simulink model "COSTEP_Exergy"  (R2024b)
settings: Solver=FixedStepAuto  StartTime=0.0  StopTime=25  FixedStep=1/3600  RelTol=1e-3
model workspace (MAT data in the model file):
  AD : Simulink.Parameter (value not decoded)
  AG : Simulink.Parameter (value not decoded)
  AH : Simulink.Parameter (value not decoded)
  AV : Simulink.Parameter (value not decoded)
  AVP : Simulink.Parameter (value not decoded)
  BCHL : Simulink.Parameter (value not decoded)
  BCHV : Simulink.Parameter (value not decoded)
  BD : Simulink.Parameter (value not decoded)
  BDIST : Simulink.Parameter (value not decoded)
  BG : Simulink.Parameter (value not decoded)
  BH : Simulink.Parameter (value not decoded)
  BVP : Simulink.Parameter (value not decoded)
  CD : Simulink.Parameter (value not decoded)
  CDIST : Simulink.Parameter (value not decoded)
  CG : Simulink.Parameter (value not decoded)
  CH : Simulink.Parameter (value not decoded)
  CVP : Simulink.Parameter (value not decoded)
  DDIST : Simulink.Parameter (value not decoded)
  DIST_CONST : Simulink.Parameter (value not decoded)
  ISV : Simulink.Parameter (value not decoded)
  TLAST : Simulink.Parameter (value not decoded)
  TNEXT : Simulink.Parameter (value not decoded)
  XMW : Simulink.Parameter (value not decoded)
  XNS : Simulink.Parameter (value not decoded)
  XNS2 : Simulink.Parameter (value not decoded)
  XNS3 : Simulink.Parameter (value not decoded)
  XNSADD : Simulink.Parameter (value not decoded)
  XNSE : Simulink.Parameter (value not decoded)
symbols that are objects in the model workspace (value not decoded): AD, AG, AH, AV, AVP, BD, BG, BH, BVP, CD, CG, CH, CVP, XMW, XNS, XNS2, XNS3, XNSE
undefined symbols (not defined in the file or in its folder): magnitude, msgbox, SETPT, XMEAS, XMV
libraries: mylib x403, dspindex x31
(part 10 of 13)

== system COSTEP_Exergy/Subsystem1/Condenser cooling water/CCin/Subsystem3 ==
  TC : Inport
  Add : Sum  Inputs=+-
  P Water Vapour Pressure Pa : Subsystem
  P0 Pa : Constant  Value=1.01325e5
  Subsystem : Subsystem
  Subsystem1 : Subsystem
  Subsystem2 : Subsystem
  T0 K : Constant  Value=298.15
  Bph : Outport
  wires:
  P Water Vapour Pressure Pa/1(P) -> Subsystem1/3(P1)
  P0 Pa/1 -> Subsystem1/4(P0)
  Subsystem/1(h-h0 J/mol) -> Add/1
  Subsystem1/1(T0(s-s0) J/mol) -> Add/2
  T0 K/1 -> Subsystem1/2(T0), Subsystem/2(T0)
  Subsystem2/1(TK) -> Subsystem/1(T1), Subsystem1/1(T1), P Water Vapour Pressure Pa/1(TK)
  TC/1 -> Subsystem2/1(TC)
  Add/1 -> Bph/1

== system COSTEP_Exergy/Subsystem1/Condenser cooling water/CCout/Subsystem ==
  Bph : Inport
  FWS : Inport  Port=2
  Gain : Gain  Gain=1/3600
  Product : Product
  Product1 : Product
  gpm to lb/h : Constant  Value=500.72
  lb/h to lb-mol/h : Product  Inputs=*/
  lb/lb-mol : Constant  Value=18.02
  mol : Constant  Value=453.59
  mol/h : Product
  Bphm J/s : Outport  VectorParamsAs1DForOutWhenUnconnected=off
  wires:
  Product/1 -> Gain/1
  mol/1 -> mol/h/1
  mol/h/1 -> Product/2
  Bph/1 -> Product/1
  FWS/1 -> Product1/1
  gpm to lb/h/1 -> Product1/2
  Product1/1 -> lb/h to lb-mol/h/1
  lb/h to lb-mol/h/1 -> mol/h/2
  lb/lb-mol/1 -> lb/h to lb-mol/h/2
  Gain/1 -> Bphm J/s/1

== system COSTEP_Exergy/Subsystem1/Condenser cooling water/CCout/Subsystem1 ==
  T : Inport
  F : Inport  Port=2
  A : Constant  Value=9.069
  Gain : Gain  Gain=1/3600
  J/mol : Product
  Product : Product
  Product1 : Product
  gpm to lb/h : Constant  Value=500.72
  lb/h to lb-mol/h : Product  Inputs=*/
  lb/lb-mol : Constant  Value=18.02
  mol : Constant  Value=453.59
  mol/h : Product
  Q J/s : Outport  VectorParamsAs1DForOutWhenUnconnected=off
  wires:
  A/1 -> J/mol/1
  mol/1 -> mol/h/1
  lb/lb-mol/1 -> lb/h to lb-mol/h/2
  Product1/1 -> lb/h to lb-mol/h/1
  lb/h to lb-mol/h/1 -> mol/h/2
  Product/1 -> Gain/1
  gpm to lb/h/1 -> Product1/2
  Gain/1 -> Q J/s/1
  mol/h/1 -> Product/2
  J/mol/1 -> Product/1
  T/1 -> J/mol/2
  F/1 -> Product1/1

== system COSTEP_Exergy/Subsystem1/Condenser cooling water/CCout/Subsystem3 ==
  TC : Inport
  Add : Sum  Inputs=+-
  P Water Vapour Pressure Pa : Subsystem
  P0 Pa : Constant  Value=1.01325e5
  Subsystem : Subsystem
  Subsystem1 : Subsystem
  Subsystem2 : Subsystem
  T0 K : Constant  Value=298.15
  Bph : Outport
  wires:
  P Water Vapour Pressure Pa/1(P) -> Subsystem1/3(P1)
  P0 Pa/1 -> Subsystem1/4(P0)
  Subsystem/1(h-h0 J/mol) -> Add/1
  Subsystem1/1(T0(s-s0) J/mol) -> Add/2
  T0 K/1 -> Subsystem1/2(T0), Subsystem/2(T0)
  Subsystem2/1(TK) -> Subsystem/1(T1), Subsystem1/1(T1), P Water Vapour Pressure Pa/1(TK)
  TC/1 -> Subsystem2/1(TC)
  Add/1 -> Bph/1

== system COSTEP_Exergy/Subsystem1/Reactor cooling water/RCin/Subsystem ==
  Bph : Inport
  FWR : Inport  Port=2
  Gain : Gain  Gain=1/3600
  Product : Product
  Product1 : Product
  gpm to lb/h : Constant  Value=500.72
  lb/h to lb-mol/h : Product  Inputs=*/
  lb/lb-mol : Constant  Value=18.02
  mol : Constant  Value=453.59
  mol/h : Product
  Bphm J/s : Outport  VectorParamsAs1DForOutWhenUnconnected=off
  wires:
  Product/1 -> Gain/1
  mol/1 -> mol/h/1
  mol/h/1 -> Product/2
  Bph/1 -> Product/1
  FWR/1 -> Product1/1
  gpm to lb/h/1 -> Product1/2
  Product1/1 -> lb/h to lb-mol/h/1
  lb/h to lb-mol/h/1 -> mol/h/2
  lb/lb-mol/1 -> lb/h to lb-mol/h/2
  Gain/1 -> Bphm J/s/1

== system COSTEP_Exergy/Subsystem1/Reactor cooling water/RCin/Subsystem1 ==
  T : Inport
  F : Inport  Port=2
  A : Constant  Value=9.069
  Gain : Gain  Gain=1/3600
  J/mol : Product
  Product : Product
  Product1 : Product
  gpm to lb/h : Constant  Value=500.72
  lb/h to lb-mol/h : Product  Inputs=*/
  lb/lb-mol : Constant  Value=18.02
  mol : Constant  Value=453.59
  mol/h : Product
  Q J/s : Outport  VectorParamsAs1DForOutWhenUnconnected=off
  wires:
  A/1 -> J/mol/1
  mol/1 -> mol/h/1
  lb/lb-mol/1 -> lb/h to lb-mol/h/2
  Product1/1 -> lb/h to lb-mol/h/1
  lb/h to lb-mol/h/1 -> mol/h/2
  Product/1 -> Gain/1
  gpm to lb/h/1 -> Product1/2
  Gain/1 -> Q J/s/1
  mol/h/1 -> Product/2
  J/mol/1 -> Product/1
  T/1 -> J/mol/2
  F/1 -> Product1/1

== system COSTEP_Exergy/Subsystem1/Reactor cooling water/RCin/Subsystem3 ==
  TC : Inport
  Add : Sum  Inputs=+-
  P Water Vapour Pressure Pa : Subsystem
  P0 Pa : Constant  Value=1.01325e5
  Subsystem : Subsystem
  Subsystem1 : Subsystem
  Subsystem2 : Subsystem
  T0 K : Constant  Value=298.15
  Bph : Outport
  wires:
  P Water Vapour Pressure Pa/1(P) -> Subsystem1/3(P1)
  P0 Pa/1 -> Subsystem1/4(P0)
  Subsystem/1(h-h0 J/mol) -> Add/1
  Subsystem1/1(T0(s-s0) J/mol) -> Add/2
  T0 K/1 -> Subsystem1/2(T0), Subsystem/2(T0)
  Subsystem2/1(TK) -> Subsystem/1(T1), Subsystem1/1(T1), P Water Vapour Pressure Pa/1(TK)
  TC/1 -> Subsystem2/1(TC)
  Add/1 -> Bph/1

== system COSTEP_Exergy/Subsystem1/Reactor cooling water/RCout/Subsystem ==
  Bph : Inport
  FWR : Inport  Port=2
  Gain : Gain  Gain=1/3600
  Product : Product
  Product1 : Product
  gpm to lb/h : Constant  Value=500.72
  lb/h to lb-mol/h : Product  Inputs=*/
  lb/lb-mol : Constant  Value=18.02
  mol : Constant  Value=453.59
  mol/h : Product
  Bphm J/s : Outport  VectorParamsAs1DForOutWhenUnconnected=off
  wires:
  Product/1 -> Gain/1
  mol/1 -> mol/h/1
  mol/h/1 -> Product/2
  Bph/1 -> Product/1
  FWR/1 -> Product1/1
  gpm to lb/h/1 -> Product1/2
  Product1/1 -> lb/h to lb-mol/h/1
  lb/h to lb-mol/h/1 -> mol/h/2
  lb/lb-mol/1 -> lb/h to lb-mol/h/2
  Gain/1 -> Bphm J/s/1

== system COSTEP_Exergy/Subsystem1/Reactor cooling water/RCout/Subsystem1 ==
  T : Inport
  F : Inport  Port=2
  A : Constant  Value=9.069
  Gain : Gain  Gain=1/3600
  J/mol : Product
  Product : Product
  Product1 : Product
  gpm to lb/h : Constant  Value=500.72
  lb/h to lb-mol/h : Product  Inputs=*/
  lb/lb-mol : Constant  Value=18.02
  mol : Constant  Value=453.59
  mol/h : Product
  Q J/s : Outport  VectorParamsAs1DForOutWhenUnconnected=off
  wires:
  A/1 -> J/mol/1
  mol/1 -> mol/h/1
  lb/lb-mol/1 -> lb/h to lb-mol/h/2
  Product1/1 -> lb/h to lb-mol/h/1
  lb/h to lb-mol/h/1 -> mol/h/2
  Product/1 -> Gain/1
  gpm to lb/h/1 -> Product1/2
  Gain/1 -> Q J/s/1
  mol/h/1 -> Product/2
  J/mol/1 -> Product/1
  T/1 -> J/mol/2
  F/1 -> Product1/1

== system COSTEP_Exergy/Subsystem1/Reactor cooling water/RCout/Subsystem3 ==
  TC : Inport
  Add : Sum  Inputs=+-
  P Water Vapour Pressure Pa : Subsystem
  P0 Pa : Constant  Value=1.01325e5
  Subsystem : Subsystem
  Subsystem1 : Subsystem
  Subsystem2 : Subsystem
  T0 K : Constant  Value=298.15
  Bph : Outport
  wires:
  P Water Vapour Pressure Pa/1(P) -> Subsystem1/3(P1)
  P0 Pa/1 -> Subsystem1/4(P0)
  Subsystem/1(h-h0 J/mol) -> Add/1
  Subsystem1/1(T0(s-s0) J/mol) -> Add/2
  T0 K/1 -> Subsystem1/2(T0), Subsystem/2(T0)
  Subsystem2/1(TK) -> Subsystem/1(T1), Subsystem1/1(T1), P Water Vapour Pressure Pa/1(TK)
  TC/1 -> Subsystem2/1(TC)
  Add/1 -> Bph/1

== system COSTEP_Exergy/Control Mode/Braatz/ /CONTROL 14/PI Control Setpoint Velocity form ==
  Setpoint : Inport
  Measurement : Inport  Port=2
  Gain : Gain  Gain=H/100
  Subsystem : Subsystem  mask{Kc=Kc, Ti=Ti, Ts=Ts, HS=HS}
      mask prompts: Kc "Controller Gain - Kc"; Ti "Integral Time - Ti"; Ts "Sampling Interval - Ts"; HS "High limit of setpoint"
      mask DialogControl DescGroupVar Prompt: Control Parameters
  Sum : Sum  Inputs=|++  SaturateOnIntegerOverflow=on
  Unit Delay : UnitDelay  InitialCondition=X_0  SampleTime=Ts
  Output : Outport
  wires:
  Gain/1 -> Sum/1
  Subsystem/1(Delta Output) -> Gain/1
  Measurement/1 -> Subsystem/2(Measurement)
  Setpoint/1 -> Subsystem/1(Setpoint)
  Sum/1 -> Unit Delay/1, Output/1
  Unit Delay/1 -> Sum/2

== system COSTEP_Exergy/Control Mode/Braatz/ 10/CONTROL 6/P Control Velocity form ==
  Setpoint : Inport
  Measurement : Inport  Port=2
  XMEAS : Inport  Port=3
  Pressure limits : Subsystem
      mask Display: color('Blue'),disp('Pressure limits'),
  Subsystem : Subsystem  mask{Kc=Kc, Ts=Ts, H=H}
      mask prompts: Kc "Controller Gain - Kc"; Ts "Sampling Interval - Ts"; H "High limit of measurement"
      mask DialogControl DescGroupVar Prompt: Control Parameters
  Sum : Sum  Inputs=|++  SaturateOnIntegerOverflow=on
  Unit Delay : UnitDelay  InitialCondition=X_0  SampleTime=Ts
  Output : Outport
  wires:
  Unit Delay/1 -> Output/1, Sum/2
  Sum/1 -> Pressure limits/1("XMV(6) ")
  Setpoint/1 -> Subsystem/1(Setpoint)
  Pressure limits/1(XMV(6)) -> Unit Delay/1
  Subsystem/1(Delta Output) -> Sum/1
  Measurement/1 -> Subsystem/2(Measurement)
  XMEAS/1 -> Pressure limits/2(XMEAS)

== system COSTEP_Exergy/Random number generator/Stream Measurements SMEAS Gas analysis1/Gas Analysis Delay/Subsystem/If Action Subsystem ==
  Action Port : ActionPort  ActionPortLabel=if(u1 == u2)
  Constant : Constant  Value=0
  Out1 : Outport  VectorParamsAs1DForOutWhenUnconnected=off
  wires:
  Constant/1 -> Out1/1

== system COSTEP_Exergy/Random number generator/Stream Measurements SMEAS Gas analysis1/Gas Analysis Delay/Subsystem/If Action Subsystem1 ==
  In1 : Inport
  Action Port : ActionPort  ActionPortLabel=else
  Out1 : Outport  VectorParamsAs1DForOutWhenUnconnected=off
  wires:
  In1/1 -> Out1/1

== system COSTEP_Exergy/Random number generator/Stream Measurements SMEAS Gas analysis1/If Action Subsystem3/Subsystem/Stream 1 ==
  G : Inport
  Bus Creator : BusCreator  Inputs=8
  Subsystem : Subsystem
  Stream 1 : Outport
  G_NEW : Outport  Port=2
  wires:
  Subsystem/4(XMNSED) -> Bus Creator/4
  Subsystem/1(XMNSEA) -> Bus Creator/1
  G/1 -> Subsystem/1(G)
  Subsystem/8(XMNSEH) -> Bus Creator/8
  Subsystem/3(XMNSEC) -> Bus Creator/3
  Subsystem/7(XMNSEG) -> Bus Creator/7
  Subsystem/9(G_NEW) -> G_NEW/1
  Subsystem/2(XMNSEB) -> Bus Creator/2
  Subsystem/5(XMNSEE) -> Bus Creator/5
  Subsystem/6(XMNSEF) -> Bus Creator/6
  Bus Creator/1 -> Stream 1/1  "Stream 1"

== system COSTEP_Exergy/Random number generator/Stream Measurements SMEAS Gas analysis1/If Action Subsystem3/Subsystem/Stream 13 ==
  G : Inport
  Bus Creator : BusCreator  Inputs=8
  Subsystem : Subsystem
  Stream 13 : Outport
  G_NEW : Outport  Port=2
  wires:
  Subsystem/4(XMNSED) -> Bus Creator/4
  Subsystem/1(XMNSEA) -> Bus Creator/1
  G/1 -> Subsystem/1(G)
  Subsystem/8(XMNSEH) -> Bus Creator/8
  Subsystem/3(XMNSEC) -> Bus Creator/3
  Subsystem/7(XMNSEG) -> Bus Creator/7
  Subsystem/9(G_NEW) -> G_NEW/1
  Subsystem/2(XMNSEB) -> Bus Creator/2
  Subsystem/5(XMNSEE) -> Bus Creator/5
  Subsystem/6(XMNSEF) -> Bus Creator/6
  Bus Creator/1 -> Stream 13/1  "Stream 13"

== system COSTEP_Exergy/Random number generator/Stream Measurements SMEAS Gas analysis1/If Action Subsystem3/Subsystem/Stream 2 ==
  G : Inport
  Bus Creator : BusCreator  Inputs=8
  Subsystem : Subsystem
  Stream 2 : Outport
  G_NEW : Outport  Port=2
  wires:
  Subsystem/4(XMNSED) -> Bus Creator/4
  Subsystem/1(XMNSEA) -> Bus Creator/1
  G/1 -> Subsystem/1(G)
  Subsystem/8(XMNSEH) -> Bus Creator/8
  Subsystem/3(XMNSEC) -> Bus Creator/3
  Subsystem/7(XMNSEG) -> Bus Creator/7
  Subsystem/9(G_NEW) -> G_NEW/1
  Subsystem/2(XMNSEB) -> Bus Creator/2
  Subsystem/5(XMNSEE) -> Bus Creator/5
  Subsystem/6(XMNSEF) -> Bus Creator/6
  Bus Creator/1 -> Stream 2/1  "Stream 2"

== system COSTEP_Exergy/Random number generator/Stream Measurements SMEAS Gas analysis1/If Action Subsystem3/Subsystem/Stream 3 ==
  G : Inport
  Bus Creator : BusCreator  Inputs=8
  Subsystem : Subsystem
  Stream 3 : Outport
  G_NEW : Outport  Port=2
  wires:
  Subsystem/4(XMNSED) -> Bus Creator/4
  Subsystem/1(XMNSEA) -> Bus Creator/1
  G/1 -> Subsystem/1(G)
  Subsystem/8(XMNSEH) -> Bus Creator/8
  Subsystem/3(XMNSEC) -> Bus Creator/3
  Subsystem/7(XMNSEG) -> Bus Creator/7
  Subsystem/9(G_NEW) -> G_NEW/1
  Subsystem/2(XMNSEB) -> Bus Creator/2
  Subsystem/5(XMNSEE) -> Bus Creator/5
  Subsystem/6(XMNSEF) -> Bus Creator/6
  Bus Creator/1 -> Stream 3/1  "Stream 3"

== system COSTEP_Exergy/Random number generator/Stream Measurements SMEAS Gas analysis1/If Action Subsystem3/Subsystem/Stream 4 ==
  G : Inport
  Bus Creator : BusCreator  Inputs=8
  Subsystem : Subsystem
  Stream 4 : Outport
  G_NEW : Outport  Port=2
  wires:
  Subsystem/4(XMNSED) -> Bus Creator/4
  Subsystem/1(XMNSEA) -> Bus Creator/1
  G/1 -> Subsystem/1(G)
  Subsystem/8(XMNSEH) -> Bus Creator/8
  Subsystem/3(XMNSEC) -> Bus Creator/3
  Subsystem/7(XMNSEG) -> Bus Creator/7
  Subsystem/9(G_NEW) -> G_NEW/1
  Subsystem/2(XMNSEB) -> Bus Creator/2
  Subsystem/5(XMNSEE) -> Bus Creator/5
  Subsystem/6(XMNSEF) -> Bus Creator/6
  Bus Creator/1 -> Stream 4/1  "Stream 4"

== system COSTEP_Exergy/Random number generator/Stream Measurements SMEAS Gas analysis1/If Action Subsystem3/Subsystem/Stream 5 ==
  G : Inport
  Bus Creator : BusCreator  Inputs=8
  Subsystem : Subsystem
  Stream 5 : Outport
  G_NEW : Outport  Port=2
  wires:
  Subsystem/4(XMNSED) -> Bus Creator/4
  Subsystem/1(XMNSEA) -> Bus Creator/1
  G/1 -> Subsystem/1(G)
  Subsystem/8(XMNSEH) -> Bus Creator/8
  Subsystem/3(XMNSEC) -> Bus Creator/3
  Subsystem/7(XMNSEG) -> Bus Creator/7
  Subsystem/9(G_NEW) -> G_NEW/1
  Subsystem/2(XMNSEB) -> Bus Creator/2
  Subsystem/5(XMNSEE) -> Bus Creator/5
  Subsystem/6(XMNSEF) -> Bus Creator/6
  Bus Creator/1 -> Stream 5/1  "Stream 5"

== system COSTEP_Exergy/Random number generator/Stream Measurements SMEAS Gas analysis1/If Action Subsystem3/Subsystem/Stream 6 ==
  G : Inport
  Bus Creator : BusCreator  Inputs=8
  Subsystem : Subsystem
  Stream 6 : Outport
  G_NEW : Outport  Port=2
  wires:
  Subsystem/4(XMNSED) -> Bus Creator/4
  Subsystem/1(XMNSEA) -> Bus Creator/1
  G/1 -> Subsystem/1(G)
  Subsystem/8(XMNSEH) -> Bus Creator/8
  Subsystem/3(XMNSEC) -> Bus Creator/3
  Subsystem/7(XMNSEG) -> Bus Creator/7
  Subsystem/9(G_NEW) -> G_NEW/1
  Subsystem/2(XMNSEB) -> Bus Creator/2
  Subsystem/5(XMNSEE) -> Bus Creator/5
  Subsystem/6(XMNSEF) -> Bus Creator/6
  Bus Creator/1 -> Stream 6/1  "Stream 6"

== system COSTEP_Exergy/Random number generator/Stream Measurements SMEAS Gas analysis1/If Action Subsystem3/Subsystem/Stream 8 ==
  G : Inport
  Bus Creator : BusCreator  Inputs=8
  Subsystem : Subsystem
  Stream 8 : Outport
  G_NEW : Outport  Port=2
  wires:
  Subsystem/4(XMNSED) -> Bus Creator/4
  Subsystem/1(XMNSEA) -> Bus Creator/1
  G/1 -> Subsystem/1(G)
  Subsystem/8(XMNSEH) -> Bus Creator/8
  Subsystem/3(XMNSEC) -> Bus Creator/3
  Subsystem/7(XMNSEG) -> Bus Creator/7
  Subsystem/9(G_NEW) -> G_NEW/1
  Subsystem/2(XMNSEB) -> Bus Creator/2
  Subsystem/5(XMNSEE) -> Bus Creator/5
  Subsystem/6(XMNSEF) -> Bus Creator/6
  Bus Creator/1 -> Stream 8/1  "Stream 8"

== system COSTEP_Exergy/Random number generator/Stream Measurements SMEAS Gas analysis1/If Action Subsystem3/Subsystem/Stream 9 ==
  G : Inport
  Bus Creator : BusCreator  Inputs=8
  Subsystem : Subsystem
  Stream 9 : Outport
  G_NEW : Outport  Port=2
  wires:
  Subsystem/4(XMNSED) -> Bus Creator/4
  Subsystem/1(XMNSEA) -> Bus Creator/1
  G/1 -> Subsystem/1(G)
  Subsystem/8(XMNSEH) -> Bus Creator/8
  Subsystem/3(XMNSEC) -> Bus Creator/3
  Subsystem/7(XMNSEG) -> Bus Creator/7
  Subsystem/9(G_NEW) -> G_NEW/1
  Subsystem/2(XMNSEB) -> Bus Creator/2
  Subsystem/5(XMNSEE) -> Bus Creator/5
  Subsystem/6(XMNSEF) -> Bus Creator/6
  Bus Creator/1 -> Stream 9/1  "Stream 9"

== system COSTEP_Exergy/Random number generator/Stream Measurements SMEAS Product analysis1/Gas Analysis Delay/Subsystem/If Action Subsystem ==
  Action Port : ActionPort  ActionPortLabel=if(u1 == u2)
  Constant : Constant  Value=0
  Out1 : Outport  VectorParamsAs1DForOutWhenUnconnected=off
  wires:
  Constant/1 -> Out1/1

== system COSTEP_Exergy/Random number generator/Stream Measurements SMEAS Product analysis1/Gas Analysis Delay/Subsystem/If Action Subsystem1 ==
  In1 : Inport
  Action Port : ActionPort  ActionPortLabel=else
  Out1 : Outport  VectorParamsAs1DForOutWhenUnconnected=off
  wires:
  In1/1 -> Out1/1

== system COSTEP_Exergy/Random number generator/Stream Measurements SMEAS Product analysis1/If Action Subsystem3/Subsystem/Subsystem1 ==
  G : Inport
  Bus Creator : BusCreator  Inputs=5
  Subsystem : Subsystem
  Stream 11 : Outport
  G_NEW : Outport  Port=2
  wires:
  Subsystem/2(XMNSEE) -> Bus Creator/2
  G/1 -> Subsystem/1(G)
  Subsystem/6(G_NEW) -> G_NEW/1
  Subsystem/5(XMNSEH) -> Bus Creator/5
  Subsystem/4(XMNSEG) -> Bus Creator/4
  Subsystem/3(XMNSEF) -> Bus Creator/3
  Subsystem/1(XMNSED) -> Bus Creator/1
  Bus Creator/1 -> Stream 11/1  "Stream 11"

== system COSTEP_Exergy/Random number generator/Stream Measurements SMEAS Product analysis1/If Action Subsystem3/Subsystem/Subsystem2 ==
  G : Inport
  Bus Creator : BusCreator  Inputs=5
  Subsystem : Subsystem
  Stream 13 : Outport
  G_NEW : Outport  Port=2
  wires:
  Subsystem/2(XMNSEE) -> Bus Creator/2
  G/1 -> Subsystem/1(G)
  Subsystem/6(G_NEW) -> G_NEW/1
  Subsystem/5(XMNSEH) -> Bus Creator/5
  Subsystem/4(XMNSEG) -> Bus Creator/4
  Subsystem/3(XMNSEF) -> Bus Creator/3
  Subsystem/1(XMNSED) -> Bus Creator/1
  Bus Creator/1 -> Stream 13/1  "Stream 13"

== system COSTEP_Exergy/Reactor/Reaction Rates/Reaction rates lb-mol//h/Reaction rate of reaction 1 lb-mol//ft3·h/If Action Subsystem ==
  In1 : Inport
  Action Port : ActionPort  ActionPortLabel=if( u1>0 & u2>0 )
  Out1 : Outport  VectorParamsAs1DForOutWhenUnconnected=off
  wires:
  In1/1 -> Out1/1

== system COSTEP_Exergy/Reactor/Reaction Rates/Reaction rates lb-mol//h/Reaction rate of reaction 1 lb-mol//ft3·h/If Action Subsystem2 ==
  In1 : Inport
  Action Port : ActionPort  ActionPortLabel=else
  Out1 : Outport  VectorParamsAs1DForOutWhenUnconnected=off
  wires:
  In1/1 -> Out1/1

== system COSTEP_Exergy/Reactor/Reaction Rates/Reaction rates lb-mol//h/Reaction rate of reaction 1 lb-mol//ft3·h/RR(1) Reaction rate of 1st reaction lb-mol//ft3·h  ==
  PPR : Inport
  TKR : Inport  Port=2
  "   " : Constant  Value=1.1544
  "    " : Constant  Value=0.3735
  Abs : Abs  SaturateOnIntegerOverflow=off
  Abs1 : Abs  SaturateOnIntegerOverflow=off
  Activation energy cal/mol : Constant  Value=40000
  Bus Selector : BusSelector  OutputSignals=PPR(1),PPR(3),PPR(4)
  Bus Selector1 : BusSelector  OutputSignals=signal1.TESUB8(7)
  Divide : Product  Inputs=*//
  Divide1 : Product  Inputs=4
  Math Function1 : Math  SignedPower=on
  Preexponential factor lb-mol/ft3·h·mmHg : Constant  Value=31.5859536
  Product : Product
  R1F : Math  Operator=pow  SignedPower=on
  R2F : Math  Operator=pow  SignedPower=on
  Subtract : Sum  Inputs=+-
  Universal gas constant cal/mol·K : Constant  Value=1.987
  RR(1) : Outport  VectorParamsAs1DForOutWhenUnconnected=off
  wires:
  "    "/1 -> R2F/2
  Divide/1 -> Subtract/2
  Universal gas constant cal/mol·K/1 -> Divide/2
  "   "/1 -> R1F/2
  Preexponential factor lb-mol/ft3·h·mmHg/1 -> Subtract/1
  Activation energy cal/mol/1 -> Divide/1
  TKR/1 -> Divide/3
  Subtract/1 -> Math Function1/1
  Divide1/1 -> RR(1)/1
  Bus Selector/2 -> Abs1/1  "<PPR(3)>"
  Abs/1 -> R1F/1
  Abs1/1 -> R2F/1
  PPR/1 -> Bus Selector/1
  Bus Selector/1 -> Abs/1  "<PPR(1)>"
  R1F/1 -> Divide1/2
  R2F/1 -> Divide1/3
  Bus Selector/3 -> Divide1/4  "<PPR(4)>"
  [TESUB8] -> Bus Selector1/1
  Math Function1/1 -> Product/1
  Bus Selector1/1 -> Product/2  "<TESUB8(7)>"
  Product/1 -> Divide1/1

== system COSTEP_Exergy/Reactor/Reaction Rates/Reaction rates lb-mol//h/Reaction rate of reaction 2 lb-mol//ft3·h/If Action Subsystem ==
  In1 : Inport
  Action Port : ActionPort  ActionPortLabel=if( u1>0 & u2>0)
  Out1 : Outport  VectorParamsAs1DForOutWhenUnconnected=off
  wires:
  In1/1 -> Out1/1

== system COSTEP_Exergy/Reactor/Reaction Rates/Reaction rates lb-mol//h/Reaction rate of reaction 2 lb-mol//ft3·h/If Action Subsystem2 ==
  In1 : Inport
  Action Port : ActionPort  ActionPortLabel=else
  Out1 : Outport  VectorParamsAs1DForOutWhenUnconnected=off
  wires:
  In1/1 -> Out1/1

== system COSTEP_Exergy/Reactor/Reaction Rates/Reaction rates lb-mol//h/Reaction rate of reaction 2 lb-mol//ft3·h/RR(2) Reaction rate of 2nd reaction lb-mol//ft3·h  ==
  PPR : Inport
  TKR : Inport  Port=2
  "   " : Constant  Value=1.1544
  "    " : Constant  Value=0.3735
  Abs : Abs  SaturateOnIntegerOverflow=off
  Abs1 : Abs  SaturateOnIntegerOverflow=off
  Activation energy cal/mol : Constant  Value=20000
  Bus Selector : BusSelector  OutputSignals=PPR(1),PPR(3),PPR(5)
  Bus Selector1 : BusSelector  OutputSignals=signal1.TESUB8(8)
  Divide : Product  Inputs=*//
  Divide1 : Product  Inputs=4
  Math Function2 : Math  SignedPower=on
  Preexponential factor lb-mol/ft3·h·mmHg : Constant  Value=3.00094014
  Product : Product
  R1F : Math  Operator=pow  SignedPower=on
  R2F : Math  Operator=pow  SignedPower=on
  Subtract : Sum  Inputs=+-
  Universal gas constant cal/mol·K : Constant  Value=1.987
  RR(2) : Outport  VectorParamsAs1DForOutWhenUnconnected=off
  wires:
  "    "/1 -> R2F/2
  Divide/1 -> Subtract/2
  Universal gas constant cal/mol·K/1 -> Divide/2
  "   "/1 -> R1F/2
  Preexponential factor lb-mol/ft3·h·mmHg/1 -> Subtract/1
  Activation energy cal/mol/1 -> Divide/1
  TKR/1 -> Divide/3
  Subtract/1 -> Math Function2/1
  Divide1/1 -> RR(2)/1
  Bus Selector/2 -> Abs1/1  "<PPR(3)>"
  Abs/1 -> R1F/1
  Abs1/1 -> R2F/1
  PPR/1 -> Bus Selector/1
  Bus Selector/1 -> Abs/1  "<PPR(1)>"
  R1F/1 -> Divide1/2
  R2F/1 -> Divide1/3
  Bus Selector/3 -> Divide1/4  "<PPR(5)>"
  [TESUB8] -> Bus Selector1/1
  Product/1 -> Divide1/1
  Math Function2/1 -> Product/1
  Bus Selector1/1 -> Product/2  "<TESUB8(8)>"

== system COSTEP_Exergy/Reactor/Reactor Heat exchanger/Reactor Heat exchanger/Cooling water outlet temperature/TCWR Inlet temperature of cooling water °C  ==
  Add : Sum
  Bus Selector : BusSelector  OutputSignals=signal1.TESUB8(5)
  Bus Selector1 : BusSelector  OutputSignals=IDV(4)
  Constant : Constant  Value=5
  Product1 : Product
  TCWR : Outport  VectorParamsAs1DForOutWhenUnconnected=off
  wires:
  Constant/1 -> Product1/2
  Bus Selector/1 -> Add/1  "<TESUB8(5)>"
  Bus Selector1/1 -> Product1/1  "<IDV(4)>"
  [TESUB8] -> Bus Selector/1
  Product1/1 -> Add/2
  [IDV] -> Bus Selector1/1
  Add/1 -> TCWR/1

== system COSTEP_Exergy/Reactor/Reactor Heat exchanger/Reactor Heat exchanger/Subsystem/If Action Subsystem ==
  In1 : Inport
  Action Port : ActionPort  ActionPortLabel=if(u1 > 50)
  Out1 : Outport  VectorParamsAs1DForOutWhenUnconnected=off
  wires:
  In1/1 -> Out1/1

== system COSTEP_Exergy/Reactor/Reactor Heat exchanger/Reactor Heat exchanger/Subsystem/If Action Subsystem1 ==
  In1 : Inport
  Action Port : ActionPort  ActionPortLabel=elseif(u1 < 10)
  Out1 : Outport  VectorParamsAs1DForOutWhenUnconnected=off
  wires:
  In1/1 -> Out1/1

== system COSTEP_Exergy/Reactor/Reactor Heat exchanger/Reactor Heat exchanger/Subsystem/If Action Subsystem2 ==
  In1 : Inport
  Action Port : ActionPort  ActionPortLabel=else
  Out1 : Outport  VectorParamsAs1DForOutWhenUnconnected=off
  wires:
  In1/1 -> Out1/1

== system COSTEP_Exergy/Separator/Stream 9/Subsystem/Pressure drop/If Action Subsystem ==
  In1 : Inport
  Action Port : ActionPort  ActionPortLabel=if(u1 < 0)
  Out1 : Outport  VectorParamsAs1DForOutWhenUnconnected=off
  wires:
  In1/1 -> Out1/1

== system COSTEP_Exergy/Separator/Stream 9/Subsystem/Pressure drop/If Action Subsystem1 ==
  In1 : Inport
  Action Port : ActionPort  ActionPortLabel=else
  Out1 : Outport  VectorParamsAs1DForOutWhenUnconnected=off
  wires:
  In1/1 -> Out1/1

== system COSTEP_Exergy/Stream Measurements/Subsystem6/A and C feed stream/Composition measurement mol%/Subsystem ==
  XST : Inport
  XMNSE : Inport  Port=2
  Bus Selector : BusSelector  OutputSignals=XMNSEA,XMNSEB,XMNSEC
  Process Noise I=23-1 : mylib/Process Noise I=23-36  SystemSampleTime=-1  VariantActivationTime=update diagram  AllowFlexibleInterface=on  Latency=0  AutoFrameSizeCalculation=off
  Process Noise I=23-2 : mylib/Process Noise I=23-36  SystemSampleTime=-1  VariantActivationTime=update diagram  AllowFlexibleInterface=on  Latency=0  AutoFrameSizeCalculation=off
  Process Noise I=23-36 : mylib/Process Noise I=23-36  SystemSampleTime=-1  VariantActivationTime=update diagram  AllowFlexibleInterface=on  Latency=0  AutoFrameSizeCalculation=off
  Subsystem : Subsystem
  SMEASXA(4) : Outport  VectorParamsAs1DForOutWhenUnconnected=off
  SMEASXB(4) : Outport  Port=2  VectorParamsAs1DForOutWhenUnconnected=off
  SMEASXC(4) : Outport  Port=3  VectorParamsAs1DForOutWhenUnconnected=off
  wires:
  Process Noise I=23-36/1 -> SMEASXA(4)/1
  Process Noise I=23-1/1 -> SMEASXB(4)/1
  Bus Selector/2 -> Process Noise I=23-1/2  "<XMNSEB>"
  Process Noise I=23-2/1 -> SMEASXC(4)/1
  Bus Selector/3 -> Process Noise I=23-2/2  "<XMNSEC>"
  Bus Selector/1 -> Process Noise I=23-36/2  "<XMNSEA>"
  XST/1 -> Subsystem/1(XST)
  Subsystem/1(XCMPA) -> Process Noise I=23-36/1
  Subsystem/2(XCMPB) -> Process Noise I=23-1/1
  Subsystem/3(XCMPC) -> Process Noise I=23-2/1
  XMNSE/1 -> Bus Selector/1

== system COSTEP_Exergy/Stream Measurements/Subsystem6/A and C feed stream/Flow measurement in kg//h/XMWS Molecular weight of Stream lb//lb-mol ==
  XST : Inport
  Product : Product
  Sum of Elements : Sum  Inputs=+
  "XMW(I) Molecular weight of components lb/lb-mol " : Constant  Value=XMW
  XMWS : Outport  VectorParamsAs1DForOutWhenUnconnected=off
  wires:
  Sum of Elements/1 -> XMWS/1
  Product/1 -> Sum of Elements/1
  XST/1 -> Product/1
  "XMW(I) Molecular weight of components lb/lb-mol "/1 -> Product/2

== system COSTEP_Exergy/Stream Measurements/Subsystem6/A feed stream/Composition measurement mol%/Subsystem ==
  XST : Inport
  XMNSE : Inport  Port=2
  Bus Selector : BusSelector  OutputSignals=XMNSEA,XMNSEB
  Process Noise I=23-1 : mylib/Process Noise I=23-36  SystemSampleTime=-1  VariantActivationTime=update diagram  AllowFlexibleInterface=on  Latency=0  AutoFrameSizeCalculation=off
  Process Noise I=23-36 : mylib/Process Noise I=23-36  SystemSampleTime=-1  VariantActivationTime=update diagram  AllowFlexibleInterface=on  Latency=0  AutoFrameSizeCalculation=off
  Subsystem : Subsystem
  SMEASXA(1) : Outport  VectorParamsAs1DForOutWhenUnconnected=off
  SMEASXB(1) : Outport  Port=2  VectorParamsAs1DForOutWhenUnconnected=off
  wires:
  Process Noise I=23-36/1 -> SMEASXA(1)/1
  Process Noise I=23-1/1 -> SMEASXB(1)/1
  Bus Selector/2 -> Process Noise I=23-1/2  "<XMNSEB>"
  Bus Selector/1 -> Process Noise I=23-36/2  "<XMNSEA>"
  XST/1 -> Subsystem/1(XST)
  Subsystem/1(XCMPA) -> Process Noise I=23-36/1
  Subsystem/2(XCMPB) -> Process Noise I=23-1/1
  XMNSE/1 -> Bus Selector/1

== system COSTEP_Exergy/Stream Measurements/Subsystem6/A feed stream/Flow measurement in kg//h/XMWS Molecular weight of Stream lb//lb-mol ==
  XST : Inport
  Product : Product
  Sum of Elements : Sum  Inputs=+
  "XMW(I) Molecular weight of components lb/lb-mol " : Constant  Value=XMW
  XMWS : Outport  VectorParamsAs1DForOutWhenUnconnected=off
  wires:
  Sum of Elements/1 -> XMWS/1
  Product/1 -> Sum of Elements/1
  XST/1 -> Product/1
  "XMW(I) Molecular weight of components lb/lb-mol "/1 -> Product/2

== system COSTEP_Exergy/Stream Measurements/Subsystem6/Condenser product stream/Composition measurement mol%/Subsystem ==
  XST : Inport
  XMNSE : Inport  Port=2
  Bus Selector : BusSelector  OutputSignals=XMNSEA,XMNSEB,XMNSEC,XMNSED,XMNSEE,XMNSEF,XMNSEG,XMNSEH
  Process Noise I=23-{1..7,36} (8 alike) : mylib/Process Noise I=23-36  SystemSampleTime=-1  VariantActivationTime=update diagram  AllowFlexibleInterface=on  Latency=0  AutoFrameSizeCalculation=off
  Subsystem : Subsystem
  SMEASXA : Outport  VectorParamsAs1DForOutWhenUnconnected=off
  SMEASXB : Outport  Port=2  VectorParamsAs1DForOutWhenUnconnected=off
  SMEASXC : Outport  Port=3  VectorParamsAs1DForOutWhenUnconnected=off
  SMEASXD : Outport  Port=4  VectorParamsAs1DForOutWhenUnconnected=off
  SMEASXE : Outport  Port=5  VectorParamsAs1DForOutWhenUnconnected=off
  SMEASXF : Outport  Port=6  VectorParamsAs1DForOutWhenUnconnected=off
  SMEASXG : Outport  Port=7  VectorParamsAs1DForOutWhenUnconnected=off
  SMEASXH : Outport  Port=8  VectorParamsAs1DForOutWhenUnconnected=off
  wires:
  Process Noise I=23-36/1 -> SMEASXA/1
  Process Noise I=23-1/1 -> SMEASXB/1
  Bus Selector/2 -> Process Noise I=23-1/2  "<XMNSEB>"
  Process Noise I=23-2/1 -> SMEASXC/1
  Process Noise I=23-3/1 -> SMEASXD/1
  Process Noise I=23-4/1 -> SMEASXE/1
  Process Noise I=23-5/1 -> SMEASXF/1
  Process Noise I=23-6/1 -> SMEASXG/1
  Process Noise I=23-7/1 -> SMEASXH/1
  Bus Selector/7 -> Process Noise I=23-6/2  "<XMNSEG>"
  Bus Selector/8 -> Process Noise I=23-7/2  "<XMNSEH>"
  Bus Selector/6 -> Process Noise I=23-5/2  "<XMNSEF>"
  Bus Selector/5 -> Process Noise I=23-4/2  "<XMNSEE>"
  Bus Selector/4 -> Process Noise I=23-3/2  "<XMNSED>"
  Bus Selector/3 -> Process Noise I=23-2/2  "<XMNSEC>"
  Bus Selector/1 -> Process Noise I=23-36/2  "<XMNSEA>"
  XST/1 -> Subsystem/1(XST)
  Subsystem/1(XCMPA) -> Process Noise I=23-36/1
  Subsystem/2(XCMPB) -> Process Noise I=23-1/1
  Subsystem/3(XCMPC) -> Process Noise I=23-2/1
  Subsystem/4(XCMPD) -> Process Noise I=23-3/1
  Subsystem/5("XCMPE ") -> Process Noise I=23-4/1
  Subsystem/6("XCMPF ") -> Process Noise I=23-5/1
  Subsystem/7(XCMPG) -> Process Noise I=23-6/1
  Subsystem/8("XCMPH ") -> Process Noise I=23-7/1
  XMNSE/1 -> Bus Selector/1

== system COSTEP_Exergy/Stream Measurements/Subsystem6/Condenser product stream/Flow measurement in kg//h/XMWS Molecular weight of Stream lb//lb-mol ==
  XST : Inport
  Product : Product
  Sum of Elements : Sum  Inputs=+
  "XMW(I) Molecular weight of components lb/lb-mol " : Constant  Value=XMW
  XMWS : Outport  VectorParamsAs1DForOutWhenUnconnected=off
  wires:
  Sum of Elements/1 -> XMWS/1
  Product/1 -> Sum of Elements/1
  XST/1 -> Product/1
  "XMW(I) Molecular weight of components lb/lb-mol "/1 -> Product/2

== system COSTEP_Exergy/Stream Measurements/Subsystem6/Condenser product stream/Subsystem/TST(8a) Temperature of Stream °C  ==
  HST : Inport  PortDimensions=1
  XLR : Inport  Port=2  PortDimensions=8
  ITY : Inport  Port=3
  "AG(I) Coefficient A to determine Enthalpy MBtu/lb·°F " : Constant  Value=AG
  "AH(I) Coefficient A to determine Enthalpy MBtu/lb·°F " : Constant  Value=AH
  AV(I) Coefficient AV to determine Enthalpy MBtu/lb : Constant  Value=AV
  BG(I) Coefficient B to determine Enthalpy MBtu/lb·°F² : Constant  Value=BG
  BH(I) Coefficient B to determine Enthalpy MBtu/lb·°F² : Constant  Value=BH
  CG(I) Coefficient C to determine Enthalpy MBtu/lb·°F³ : Constant  Value=CG
  CH(I) Coefficient C to determine Enthalpy MBtu/lb·°F³ : Constant  Value=CH
  Delay : Delay  DelayLength=1  InitialCondition=0
  MATLAB Function : MATLAB Function  TreatAsAtomicUnit=on
  "XMW(I) Molecular weight of components lb/lb-mol " : Constant  Value=XMW
  TST(8a) : Outport  PortDimensions=1  VectorParamsAs1DForOutWhenUnconnected=off
  wires:
  MATLAB Function/1(TST) -> Delay/1, TST(8a)/1
  Delay/1 -> MATLAB Function/12("TST ")
  "AG(I) Coefficient A to determine Enthalpy MBtu/lb·°F "/1 -> MATLAB Function/4(AG)
  AV(I) Coefficient AV to determine Enthalpy MBtu/lb/1 -> MATLAB Function/7(AV)
  HST/1 -> MATLAB Function/10(HST)
  CH(I) Coefficient C to determine Enthalpy MBtu/lb·°F³/1 -> MATLAB Function/3(CH)
  ITY/1 -> MATLAB Function/11(ITY)
  "XMW(I) Molecular weight of components lb/lb-mol "/1 -> MATLAB Function/8(XMW)
  XLR/1 -> MATLAB Function/9(XLR)
  "AH(I) Coefficient A to determine Enthalpy MBtu/lb·°F "/1 -> MATLAB Function/1(AH)
  CG(I) Coefficient C to determine Enthalpy MBtu/lb·°F³/1 -> MATLAB Function/6(CG)
  BH(I) Coefficient B to determine Enthalpy MBtu/lb·°F²/1 -> MATLAB Function/2(BH)
  BG(I) Coefficient B to determine Enthalpy MBtu/lb·°F²/1 -> MATLAB Function/5(BG)

== system COSTEP_Exergy/Stream Measurements/Subsystem6/D feed stream/Composition measurement mol%/Subsystem ==
  XST : Inport
  XMNSE : Inport  Port=2
  Bus Selector : BusSelector  OutputSignals=XMNSEB,XMNSED
  Process Noise I=23-1 : mylib/Process Noise I=23-36  SystemSampleTime=-1  VariantActivationTime=update diagram  AllowFlexibleInterface=on  Latency=0  AutoFrameSizeCalculation=off
  Process Noise I=23-3 : mylib/Process Noise I=23-36  SystemSampleTime=-1  VariantActivationTime=update diagram  AllowFlexibleInterface=on  Latency=0  AutoFrameSizeCalculation=off
  Subsystem : Subsystem
  SMEASXB(2) : Outport  VectorParamsAs1DForOutWhenUnconnected=off
  SMEASXD(2) : Outport  Port=2  VectorParamsAs1DForOutWhenUnconnected=off
  wires:
  Process Noise I=23-1/1 -> SMEASXB(2)/1
  Bus Selector/1 -> Process Noise I=23-1/2  "<XMNSEB>"
  Process Noise I=23-3/1 -> SMEASXD(2)/1
  Bus Selector/2 -> Process Noise I=23-3/2  "<XMNSED>"
  XST/1 -> Subsystem/1(XST)
  Subsystem/1(XCMPB) -> Process Noise I=23-1/1
  Subsystem/2(XCMPD) -> Process Noise I=23-3/1
  XMNSE/1 -> Bus Selector/1

== system COSTEP_Exergy/Stream Measurements/Subsystem6/E feed stream/Composition measurement mol%/Subsystem ==
  XST : Inport
  XMNSE : Inport  Port=2
  Bus Selector : BusSelector  OutputSignals=XMNSEE,XMNSEF
  Process Noise I=23-4 : mylib/Process Noise I=23-36  SystemSampleTime=-1  VariantActivationTime=update diagram  AllowFlexibleInterface=on  Latency=0  AutoFrameSizeCalculation=off
  Process Noise I=23-5 : mylib/Process Noise I=23-36  SystemSampleTime=-1  VariantActivationTime=update diagram  AllowFlexibleInterface=on  Latency=0  AutoFrameSizeCalculation=off
  Subsystem : Subsystem
  SMEASXE(3) : Outport  VectorParamsAs1DForOutWhenUnconnected=off
  SMEASXF(3) : Outport  Port=2  VectorParamsAs1DForOutWhenUnconnected=off
  wires:
  Process Noise I=23-4/1 -> SMEASXE(3)/1
  Process Noise I=23-5/1 -> SMEASXF(3)/1
  Bus Selector/2 -> Process Noise I=23-5/2  "<XMNSEF>"
  Bus Selector/1 -> Process Noise I=23-4/2  "<XMNSEE>"
  XST/1 -> Subsystem/1(XST)
  Subsystem/1("XCMPE ") -> Process Noise I=23-4/1
  Subsystem/2("XCMPF ") -> Process Noise I=23-5/1
  XMNSE/1 -> Bus Selector/1

== system COSTEP_Exergy/Stream Measurements/Subsystem6/Product stream/Composition measurement mol%/Subsystem ==
  XST : Inport
  XMNSE : Inport  Port=2
  Bus Selector : BusSelector  OutputSignals=XMNSEA,XMNSEB,XMNSEC
  Process Noise I=23-1 : mylib/Process Noise I=23-36  SystemSampleTime=-1  VariantActivationTime=update diagram  AllowFlexibleInterface=on  Latency=0  AutoFrameSizeCalculation=off
  Process Noise I=23-2 : mylib/Process Noise I=23-36  SystemSampleTime=-1  VariantActivationTime=update diagram  AllowFlexibleInterface=on  Latency=0  AutoFrameSizeCalculation=off
  Process Noise I=23-36 : mylib/Process Noise I=23-36  SystemSampleTime=-1  VariantActivationTime=update diagram  AllowFlexibleInterface=on  Latency=0  AutoFrameSizeCalculation=off
  Subsystem : Subsystem
  SMEASXA : Outport  VectorParamsAs1DForOutWhenUnconnected=off
  SMEASXB : Outport  Port=2  VectorParamsAs1DForOutWhenUnconnected=off
  SMEASXC : Outport  Port=3  VectorParamsAs1DForOutWhenUnconnected=off
  wires:
  Process Noise I=23-36/1 -> SMEASXA/1
  Process Noise I=23-1/1 -> SMEASXB/1
  Bus Selector/2 -> Process Noise I=23-1/2  "<XMNSEB>"
  Process Noise I=23-2/1 -> SMEASXC/1
  Bus Selector/3 -> Process Noise I=23-2/2  "<XMNSEC>"
  Bus Selector/1 -> Process Noise I=23-36/2  "<XMNSEA>"
  XST/1 -> Subsystem/1(XST)
  Subsystem/1(XCMPA) -> Process Noise I=23-36/1
  Subsystem/2(XCMPB) -> Process Noise I=23-1/1
  Subsystem/3(XCMPC) -> Process Noise I=23-2/1
  XMNSE/1 -> Bus Selector/1

== system COSTEP_Exergy/Stream Measurements/Subsystem6/Product stream/Composition measurement mol%/Subsystem1 ==
  XST : Inport
  XMNSE3 : Inport  Port=2
  Bus Selector : BusSelector  OutputSignals=XMNSED,XMNSEE,XMNSEF,XMNSEG,XMNSEH
  Process Noise I=37-{1..4,41} (5 alike) : mylib/Process Noise I=37-41  SystemSampleTime=-1  VariantActivationTime=update diagram  AllowFlexibleInterface=on  Latency=0  AutoFrameSizeCalculation=off
  Subsystem : Subsystem
  SMEASXD : Outport  VectorParamsAs1DForOutWhenUnconnected=off
  SMEASXE : Outport  Port=2  VectorParamsAs1DForOutWhenUnconnected=off
  SMEASXF : Outport  Port=3  VectorParamsAs1DForOutWhenUnconnected=off
  SMEASXG : Outport  Port=4  VectorParamsAs1DForOutWhenUnconnected=off
  SMEASXH : Outport  Port=5  VectorParamsAs1DForOutWhenUnconnected=off
  wires:
  Process Noise I=37-41/1 -> SMEASXD/1
  Bus Selector/1 -> Process Noise I=37-41/2  "<XMNSED>"
  Process Noise I=37-1/1 -> SMEASXE/1
  Bus Selector/2 -> Process Noise I=37-1/2  "<XMNSEE>"
  Process Noise I=37-2/1 -> SMEASXF/1
  Bus Selector/3 -> Process Noise I=37-2/2  "<XMNSEF>"
  Process Noise I=37-3/1 -> SMEASXG/1
  Bus Selector/4 -> Process Noise I=37-3/2  "<XMNSEG>"
  Process Noise I=37-4/1 -> SMEASXH/1
  Bus Selector/5 -> Process Noise I=37-4/2  "<XMNSEH>"
  XST/1 -> Subsystem/1(XST)
  Subsystem/1(XCMPD) -> Process Noise I=37-41/1
  Subsystem/2("XCMPE ") -> Process Noise I=37-1/1
  Subsystem/3("XCMPF ") -> Process Noise I=37-2/1
  Subsystem/4(XCMPG) -> Process Noise I=37-3/1
  Subsystem/5("XCMPH ") -> Process Noise I=37-4/1
  XMNSE3/1 -> Bus Selector/1

== system COSTEP_Exergy/Stream Measurements/Subsystem6/Product stream/Flow measurement in kg//h/XMWS Molecular weight of Stream lb//lb-mol ==
  XST : Inport
  Product : Product
  Sum of Elements : Sum  Inputs=+
  "XMW(I) Molecular weight of components lb/lb-mol " : Constant  Value=XMW
  XMWS : Outport  VectorParamsAs1DForOutWhenUnconnected=off
  wires:
  Sum of Elements/1 -> XMWS/1
  Product/1 -> Sum of Elements/1
  XST/1 -> Product/1
  "XMW(I) Molecular weight of components lb/lb-mol "/1 -> Product/2

== system COSTEP_Exergy/Stream Measurements/Subsystem6/Purge stream/Flow measurement in kg//h/XMWS Molecular weight of Stream lb//lb-mol ==
  XST : Inport
  Product : Product
  Sum of Elements : Sum  Inputs=+
  "XMW(I) Molecular weight of components lb/lb-mol " : Constant  Value=XMW
  XMWS : Outport  VectorParamsAs1DForOutWhenUnconnected=off
  wires:
  Sum of Elements/1 -> XMWS/1
  Product/1 -> Sum of Elements/1
  XST/1 -> Product/1
  "XMW(I) Molecular weight of components lb/lb-mol "/1 -> Product/2

== system COSTEP_Exergy/Stream Measurements/Subsystem6/Reactor feed stream/Composition measurement mol%/Subsystem ==
  XST : Inport
  XMNSE : Inport  Port=2
  XMEAS : Inport  Port=3
  Bus Selector : BusSelector  OutputSignals=XMNSEG,XMNSEH
  Bus Selector1 : BusSelector  OutputSignals=XMEAS(23),XMEAS(24),XMEAS(25),XMEAS(26),XMEAS(27),XMEAS(28)
  Process Noise I=23-6 : mylib/Process Noise I=23-36  SystemSampleTime=-1  VariantActivationTime=update diagram  AllowFlexibleInterface=on  Latency=0  AutoFrameSizeCalculation=off
  Process Noise I=23-7 : mylib/Process Noise I=23-36  SystemSampleTime=-1  VariantActivationTime=update diagram  AllowFlexibleInterface=on  Latency=0  AutoFrameSizeCalculation=off
  Subsystem : Subsystem
  SMEASXA : Outport  VectorParamsAs1DForOutWhenUnconnected=off
  SMEASXB : Outport  Port=2  VectorParamsAs1DForOutWhenUnconnected=off
  SMEASXC : Outport  Port=3  VectorParamsAs1DForOutWhenUnconnected=off
  SMEASXD : Outport  Port=4  VectorParamsAs1DForOutWhenUnconnected=off
  SMEASXE : Outport  Port=5  VectorParamsAs1DForOutWhenUnconnected=off
  SMEASXF : Outport  Port=6  VectorParamsAs1DForOutWhenUnconnected=off
  SMEASXG : Outport  Port=7  VectorParamsAs1DForOutWhenUnconnected=off
  SMEASXH : Outport  Port=8  VectorParamsAs1DForOutWhenUnconnected=off
  wires:
  Bus Selector1/1 -> SMEASXA/1  "<XMEAS(23)>"
  Bus Selector1/2 -> SMEASXB/1  "<XMEAS(24)>"
  Bus Selector1/3 -> SMEASXC/1  "<XMEAS(25)>"
  Bus Selector1/4 -> SMEASXD/1  "<XMEAS(26)>"
  Bus Selector1/5 -> SMEASXE/1  "<XMEAS(27)>"
  Bus Selector1/6 -> SMEASXF/1  "<XMEAS(28)>"
  Process Noise I=23-6/1 -> SMEASXG/1
  Process Noise I=23-7/1 -> SMEASXH/1
  Bus Selector/1 -> Process Noise I=23-6/2  "<XMNSEG>"
  Bus Selector/2 -> Process Noise I=23-7/2  "<XMNSEH>"
  XST/1 -> Subsystem/1(XST)
  Subsystem/1(XCMPG) -> Process Noise I=23-6/1
  Subsystem/2("XCMPH ") -> Process Noise I=23-7/1
  XMNSE/1 -> Bus Selector/1
  XMEAS/1 -> Bus Selector1/1

== system COSTEP_Exergy/Stream Measurements/Subsystem6/Reactor feed stream/Flow measurement in kg//h/XMWS Molecular weight of Stream lb//lb-mol ==
  XST : Inport
  Product : Product
  Sum of Elements : Sum  Inputs=+
  "XMW(I) Molecular weight of components lb/lb-mol " : Constant  Value=XMW
  XMWS : Outport  VectorParamsAs1DForOutWhenUnconnected=off
  wires:
  Sum of Elements/1 -> XMWS/1
  Product/1 -> Sum of Elements/1
  XST/1 -> Product/1
  "XMW(I) Molecular weight of components lb/lb-mol "/1 -> Product/2

== system COSTEP_Exergy/Stream Measurements/Subsystem6/Reactor product stream/Composition measurement mol%/Subsystem ==
  XST : Inport
  XMNSE : Inport  Port=2
  Bus Selector : BusSelector  OutputSignals=XMNSEA,XMNSEB,XMNSEC,XMNSED,XMNSEE,XMNSEF,XMNSEG,XMNSEH
  Process Noise I=23-{1..7,36} (8 alike) : mylib/Process Noise I=23-36  SystemSampleTime=-1  VariantActivationTime=update diagram  AllowFlexibleInterface=on  Latency=0  AutoFrameSizeCalculation=off
  Subsystem : Subsystem
  SMEASXA(7) : Outport  VectorParamsAs1DForOutWhenUnconnected=off
  SMEASXB(7) : Outport  Port=2  VectorParamsAs1DForOutWhenUnconnected=off
  SMEASXC(7) : Outport  Port=3  VectorParamsAs1DForOutWhenUnconnected=off
  SMEASXD(7) : Outport  Port=4  VectorParamsAs1DForOutWhenUnconnected=off
  SMEASXE(7) : Outport  Port=5  VectorParamsAs1DForOutWhenUnconnected=off
  SMEASXF(7) : Outport  Port=6  VectorParamsAs1DForOutWhenUnconnected=off
  SMEASXG(7) : Outport  Port=7  VectorParamsAs1DForOutWhenUnconnected=off
  SMEASXH(7) : Outport  Port=8  VectorParamsAs1DForOutWhenUnconnected=off
  wires:
  Process Noise I=23-36/1 -> SMEASXA(7)/1
  Process Noise I=23-1/1 -> SMEASXB(7)/1
  Bus Selector/2 -> Process Noise I=23-1/2  "<XMNSEB>"
  Process Noise I=23-2/1 -> SMEASXC(7)/1
  Process Noise I=23-3/1 -> SMEASXD(7)/1
  Process Noise I=23-4/1 -> SMEASXE(7)/1
  Process Noise I=23-5/1 -> SMEASXF(7)/1
  Process Noise I=23-6/1 -> SMEASXG(7)/1
  Process Noise I=23-7/1 -> SMEASXH(7)/1
  Bus Selector/7 -> Process Noise I=23-6/2  "<XMNSEG>"
  Bus Selector/8 -> Process Noise I=23-7/2  "<XMNSEH>"
  Bus Selector/6 -> Process Noise I=23-5/2  "<XMNSEF>"
  Bus Selector/5 -> Process Noise I=23-4/2  "<XMNSEE>"
  Bus Selector/4 -> Process Noise I=23-3/2  "<XMNSED>"
  Bus Selector/3 -> Process Noise I=23-2/2  "<XMNSEC>"
  Bus Selector/1 -> Process Noise I=23-36/2  "<XMNSEA>"
  XST/1 -> Subsystem/1(XST)
  Subsystem/1(XCMPA) -> Process Noise I=23-36/1
  Subsystem/2(XCMPB) -> Process Noise I=23-1/1
  Subsystem/3(XCMPC) -> Process Noise I=23-2/1
  Subsystem/4(XCMPD) -> Process Noise I=23-3/1
  Subsystem/5("XCMPE ") -> Process Noise I=23-4/1
  Subsystem/6("XCMPF ") -> Process Noise I=23-5/1
  Subsystem/7(XCMPG) -> Process Noise I=23-6/1
  Subsystem/8("XCMPH ") -> Process Noise I=23-7/1
  XMNSE/1 -> Bus Selector/1

== system COSTEP_Exergy/Stream Measurements/Subsystem6/Reactor product stream/Flow measurement in kg//h/XMWS Molecular weight of Stream lb//lb-mol ==
  XST : Inport
  Product : Product
  Sum of Elements : Sum  Inputs=+
  "XMW(I) Molecular weight of components lb/lb-mol " : Constant  Value=XMW
  XMWS : Outport  VectorParamsAs1DForOutWhenUnconnected=off
  wires:
  Sum of Elements/1 -> XMWS/1
  Product/1 -> Sum of Elements/1
  XST/1 -> Product/1
  "XMW(I) Molecular weight of components lb/lb-mol "/1 -> Product/2

== system COSTEP_Exergy/Stream Measurements/Subsystem6/Separator product stream/Composition measurement mol%/Subsystem ==
  XST : Inport
  XMNSE : Inport  Port=2
  Bus Selector : BusSelector  OutputSignals=XMNSEA,XMNSEB,XMNSEC,XMNSED,XMNSEE,XMNSEF,XMNSEG,XMNSEH
  Process Noise I=23-{1..7,36} (8 alike) : mylib/Process Noise I=23-36  SystemSampleTime=-1  VariantActivationTime=update diagram  AllowFlexibleInterface=on  Latency=0  AutoFrameSizeCalculation=off
  Subsystem : Subsystem
  SMEASXA : Outport  VectorParamsAs1DForOutWhenUnconnected=off
  SMEASXB : Outport  Port=2  VectorParamsAs1DForOutWhenUnconnected=off
  SMEASXC : Outport  Port=3  VectorParamsAs1DForOutWhenUnconnected=off
  SMEASXD : Outport  Port=4  VectorParamsAs1DForOutWhenUnconnected=off
  SMEASXE : Outport  Port=5  VectorParamsAs1DForOutWhenUnconnected=off
  SMEASXF : Outport  Port=6  VectorParamsAs1DForOutWhenUnconnected=off
  SMEASXG : Outport  Port=7  VectorParamsAs1DForOutWhenUnconnected=off
  SMEASXH : Outport  Port=8  VectorParamsAs1DForOutWhenUnconnected=off
  wires:
  Process Noise I=23-36/1 -> SMEASXA/1
  Process Noise I=23-1/1 -> SMEASXB/1
  Bus Selector/2 -> Process Noise I=23-1/2  "<XMNSEB>"
  Process Noise I=23-2/1 -> SMEASXC/1
  Process Noise I=23-3/1 -> SMEASXD/1
  Process Noise I=23-4/1 -> SMEASXE/1
  Process Noise I=23-5/1 -> SMEASXF/1
  Process Noise I=23-6/1 -> SMEASXG/1
  Process Noise I=23-7/1 -> SMEASXH/1
  Bus Selector/7 -> Process Noise I=23-6/2  "<XMNSEG>"
  Bus Selector/8 -> Process Noise I=23-7/2  "<XMNSEH>"
  Bus Selector/6 -> Process Noise I=23-5/2  "<XMNSEF>"
  Bus Selector/5 -> Process Noise I=23-4/2  "<XMNSEE>"
  Bus Selector/4 -> Process Noise I=23-3/2  "<XMNSED>"
  Bus Selector/3 -> Process Noise I=23-2/2  "<XMNSEC>"
  Bus Selector/1 -> Process Noise I=23-36/2  "<XMNSEA>"
  XST/1 -> Subsystem/1(XST)
  Subsystem/1(XCMPA) -> Process Noise I=23-36/1
  Subsystem/2(XCMPB) -> Process Noise I=23-1/1
  Subsystem/3(XCMPC) -> Process Noise I=23-2/1
  Subsystem/4(XCMPD) -> Process Noise I=23-3/1
  Subsystem/5("XCMPE ") -> Process Noise I=23-4/1
  Subsystem/6("XCMPF ") -> Process Noise I=23-5/1
  Subsystem/7(XCMPG) -> Process Noise I=23-6/1
  Subsystem/8("XCMPH ") -> Process Noise I=23-7/1
  XMNSE/1 -> Bus Selector/1

== system COSTEP_Exergy/Stream Measurements/Subsystem6/Separator product stream/Flow measurement in kg//h/Subsystem ==
  XST : Inport
  XMEAS : Inport  Port=2
  " " : Constant  Value=35.3145
  "  " : Constant  Value=0.359
  Convert from lb/h to kg/h : Constant  Value=0.454
  Product : Product  Inputs=3
  XMWS Molecular weight of Stream lb/lb-mol : Subsystem
  lb-mol/h : Product  Inputs=**/
  SMEAS F : Outport
  wires:
  lb-mol/h/1 -> Product/2
  " "/1 -> lb-mol/h/2
  XST/1 -> XMWS Molecular weight of Stream lb/lb-mol/1(XST)
  "  "/1 -> lb-mol/h/3
  Product/1 -> SMEAS F/1
  Convert from lb/h to kg/h/1 -> Product/3
  XMWS Molecular weight of Stream lb/lb-mol/1(XMWS) -> Product/1
  XMEAS/1 -> lb-mol/h/1

== system COSTEP_Exergy/Stream Measurements/Subsystem6/Separator product stream/Flow measurement in kg//h/Subsystem1 ==
  XST : Inport
  XMEAS : Inport  Port=2
  " " : Constant  Value=35.3145
  "  " : Constant  Value=0.359
  Convert from lb/h to kg/h : Constant  Value=0.454
  Product : Product  Inputs=3
  XMWS Molecular weight of Stream lb/lb-mol : Subsystem
  lb-mol/h : Product  Inputs=**/
  SMEAS F : Outport
  wires:
  lb-mol/h/1 -> Product/2
  " "/1 -> lb-mol/h/2
  XST/1 -> XMWS Molecular weight of Stream lb/lb-mol/1(XST)
  "  "/1 -> lb-mol/h/3
  Product/1 -> SMEAS F/1
  Convert from lb/h to kg/h/1 -> Product/3
  XMWS Molecular weight of Stream lb/lb-mol/1(XMWS) -> Product/1
  XMEAS/1 -> lb-mol/h/1
